simulink model "model2f"  (R2020a)
settings: Solver=VariableStepAuto  StartTime=0.0  StopTime=10.0  RelTol=1e-3
values from neighbouring files (symbols this model uses):
  A = [ ... (first row only)    [a2p1.m]    (also in p1.m; p2f.m; p2g.m)
  B = [0; 0; 0; 0; 7.5]    [p2f.m]    (also in p2g.m = [0; 0; 0; 0; 7.5;])
  C = [ 1 0 0 0 0 ... (first row only)    [p2f.m]    (also in p2g.m)
  d = 1.5*pi/180    (= 0.0261799387799)    [a2p2.m]    (also in p2c_e.m; p2f.m; p2g.m)
  D = zeros(4,1)    [p2f.m]    (also in p2g.m)
  g = 9.81    [a2p2.m]    (also in p2c_e.m; p2f.m; p2g.m)
  kd_phi = (2*zeta_phi*omega_n_phi - a_phi1)/a_phi2    [a2p2.m]    (also in p2c.m = 2.24; p2c_e.m; p2f.m; p2g.m)
  ki_chi = (omega_n_chi)^2 * V_g/g    [a2p2.m]    (also in p2c_e.m; p2f.m; p2g.m)
  kp_chi = 2*zeta_chi*omega_n_chi*V_g/g    [a2p2.m]    (also in p2c_e.m; p2f.m; p2g.m)
  kp_phi = (delta_max_a/e_max_a)*sign(a_phi2)    [a2p2.m]    (also in p2c.m = delta_max / e_phimax * sign(a_phi2); p2c_e.m; p2f.m; p2g.m)
  V_g = V_a    (= 580)    [a2p2.m]    (also in p2c_e.m; p2f.m; p2g.m)
libraries: simulink_extras x3
settings Model: Creator=ivermyklebust  LastModifiedBy=ivermyklebust

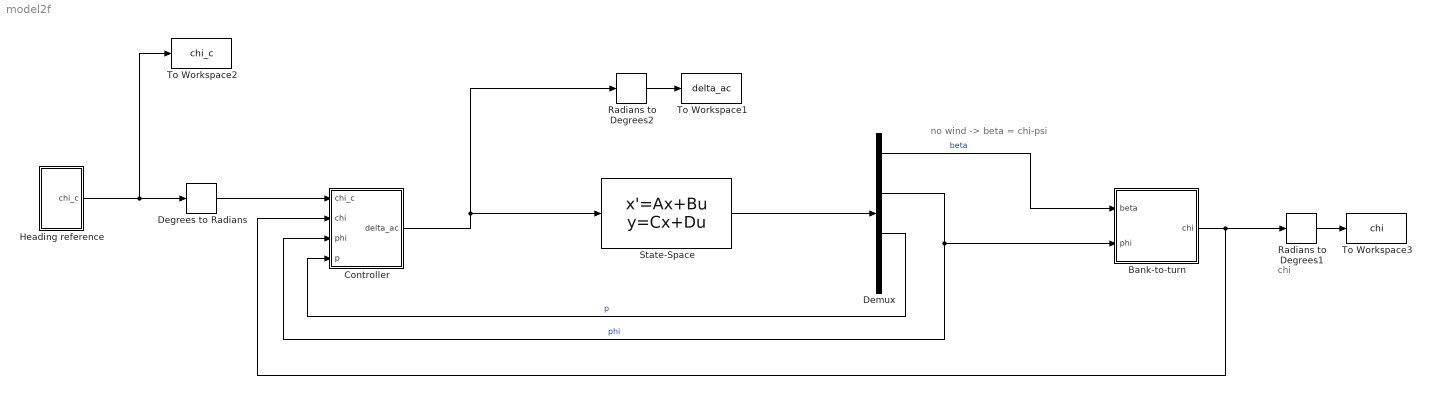
== system model2f ==
  note: no wind -> beta = chi-psi
  note: chi
  Bank-to-turn : Subsystem
  Controller : Subsystem
  Degrees to Radians : simulink_extras/Transformations/Degrees to Radians
  Demux : Demux
  Heading reference : Subsystem
  Radians to Degrees1 : simulink_extras/Transformations/Radians to Degrees
  Radians to Degrees2 : simulink_extras/Transformations/Radians to Degrees
  State-Space : StateSpace  A=A  B=B  C=C  D=D  InitialCondition=0
  To Workspace1 : ToWorkspace  VariableName=delta_ac  SaveFormat=Timeseries  SampleTime=-1
  To Workspace2 : ToWorkspace  VariableName=chi_c  SaveFormat=Timeseries  SampleTime=-1
  To Workspace3 : ToWorkspace  VariableName=chi  SaveFormat=Timeseries  SampleTime=-1
  wires:
  Radians to Degrees1/1 -> To Workspace3/1
  Demux/2 -> Controller/3(phi), Bank-to-turn/2(phi)  "phi"
  Radians to Degrees2/1 -> To Workspace1/1
  State-Space/1 -> Demux/1
  Heading reference/1(chi_c) -> To Workspace2/1, Degrees to Radians/1
  Bank-to-turn/1(chi) -> Controller/2(chi), Radians to Degrees1/1
  Demux/1 -> Bank-to-turn/1(beta)  "beta"
  Controller/1(delta_ac) -> Radians to Degrees2/1, State-Space/1
  Degrees to Radians/1 -> Controller/1(chi_c)
  Demux/3 -> Controller/4(p)  "p"

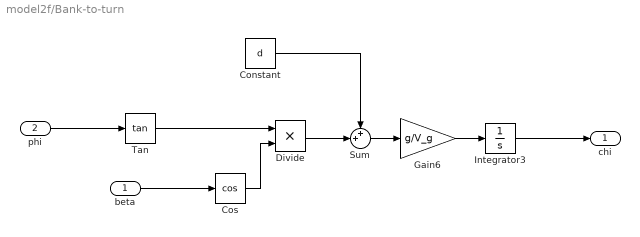
== system model2f/Bank-to-turn ==
  beta : Inport
  phi : Inport  Port=2
  Constant : Constant  Value=d
  Cos : Trigonometry  Operator=cos
  Divide : Product  Inputs=**
  Gain6 : Gain  Gain=g/V_g
  Integrator3 : Integrator
  Sum : Sum  Inputs=++|
  Tan : Trigonometry  Operator=tan
  chi : Outport
  wires:
  phi/1 -> Tan/1
  Tan/1 -> Divide/1
  Cos/1 -> Divide/2
  Integrator3/1 -> chi/1
  beta/1 -> Cos/1
  Gain6/1 -> Integrator3/1
  Constant/1 -> Sum/1
  Sum/1 -> Gain6/1
  Divide/1 -> Sum/2

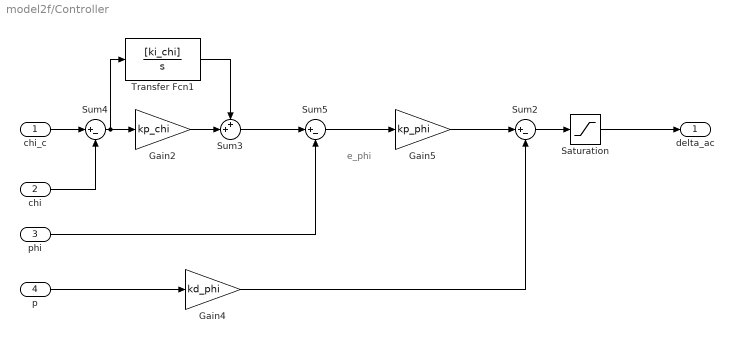
== system model2f/Controller ==
  note: e_phi
  chi_c : Inport
  chi : Inport  Port=2
  phi : Inport  Port=3
  p : Inport  Port=4
  Gain2 : Gain  Gain=kp_chi
  Gain4 : Gain  Gain=kd_phi
  Gain5 : Gain  Gain=kp_phi
  Saturation : Saturate  UpperLimit=pi/6  LowerLimit=-pi/6
  Sum2 : Sum  Inputs=|+-
  Sum3 : Sum  Inputs=++|
  Sum4 : Sum  Inputs=|+-
  Sum5 : Sum  Inputs=|+-
  Transfer Fcn1 : TransferFcn  Numerator=[ki_chi]  Denominator=[1 0]
  delta_ac : Outport
  wires:
  Sum4/1 -> Transfer Fcn1/1, Gain2/1
  chi/1 -> Sum4/2
  p/1 -> Gain4/1
  Gain2/1 -> Sum3/2
  Gain5/1 -> Sum2/1
  Saturation/1 -> delta_ac/1
  chi_c/1 -> Sum4/1
  phi/1 -> Sum5/2
  Sum2/1 -> Saturation/1
  Sum5/1 -> Gain5/1
  Sum3/1 -> Sum5/1
  Transfer Fcn1/1 -> Sum3/1
  Gain4/1 -> Sum2/2

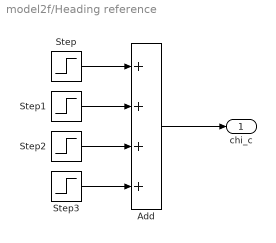
== system model2f/Heading reference ==
  Add : Sum  Inputs=++++
  Step : Step  Time=100  After=7.5  SampleTime=0
  Step1 : Step  Time=200  After=7.5  SampleTime=0
  Step2 : Step  Time=300  After=-7.5  SampleTime=0
  Step3 : Step  Time=400  After=0  SampleTime=0
  chi_c : Outport
  wires:
  Step2/1 -> Add/3
  Add/1 -> chi_c/1
  Step3/1 -> Add/4
  Step1/1 -> Add/2
  Step/1 -> Add/1
